simulink model "Hydraulic787"  (R2013a)
settings: Solver=ode23tb  StartTime=0.0  StopTime=1000  RelTol=1e-3
InitFcn:
  | load('SampleOutput.mat')
  | 
  | load('SampleFuelBurn.mat')
undefined symbols (not defined in the file): ailerons, AirProp, B_737, elevator, HydProp, landing_gear, rudder, thrust_rev
libraries: PowerFlowLib x43, simulink x4
(part 1 of 2)
settings Model: Creator=ASELab1  LastModifiedBy=ASELab1
settings SolverCC: SolverJacobianMethodControl=FullAnalytical

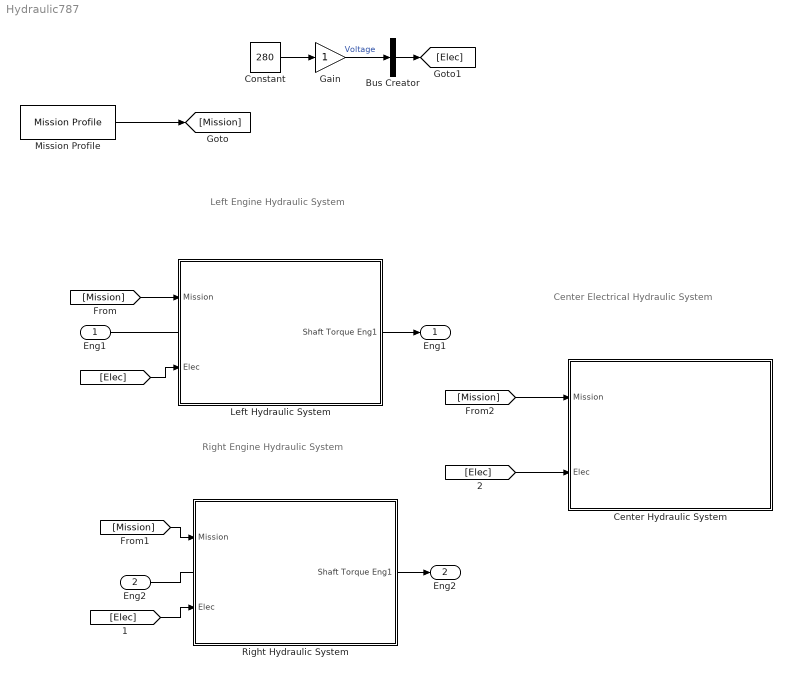
== system Hydraulic787 ==
  note: Left Engine Hydraulic System
  note: Right Engine Hydraulic System
  note: Center Electrical Hydraulic System
  Eng1 : Inport
  Eng2 : Inport  Port=2
  Bus Creator : BusCreator  Inputs=1
  Center Hydraulic System : Subsystem  mask{Hyd_Pump_Pres=34473.79}
      mask prompts: Hyd_Pump_Pres "Hyrdaulic Pump Pressure (kpa)"
  Constant : Constant  Value=280
  Gain : Gain
  Left Hydraulic System : Subsystem  mask{Hyd_Pump_Pres=34473.79}
      mask prompts: Hyd_Pump_Pres "Hyrdaulic Pump Pressure (kpa)"
  Mission Profile : PowerFlowLib/Mission Profile/Mission Profile  mssn_check=off  mssn_prof=MSSN  del_P=0  del_T=0  del_rho=0  pres_msl=101.3  temp_msl=15  dens_msl=1.229
  Right Hydraulic System : Subsystem  mask{Hyd_Pump_Pres=34473.79}
      mask prompts: Hyd_Pump_Pres "Hyrdaulic Pump Pressure (kpa)"
  "Eng1 " : Outport
  "Eng2 " : Outport  Port=2
  wires:
  Mission Profile/1 -> [Mission]
  Eng1/1 -> ?
  [Mission] -> Right Hydraulic System/1(Mission)
  [Mission] -> Center Hydraulic System/1(Mission)
  [Mission] -> Left Hydraulic System/1(Mission)
  Eng2/1 -> ?
  Left Hydraulic System/1(Shaft Torque Eng1) -> "Eng1 "/1
  Right Hydraulic System/1(Shaft Torque Eng1) -> "Eng2 "/1
  [Elec] -> Center Hydraulic System/2(Elec)
  [Elec] -> Left Hydraulic System/2(Elec)
  [Elec] -> Right Hydraulic System/2(Elec)
  Constant/1 -> Gain/1
  Bus Creator/1 -> [Elec]
  Gain/1 -> Bus Creator/1  "Voltage"

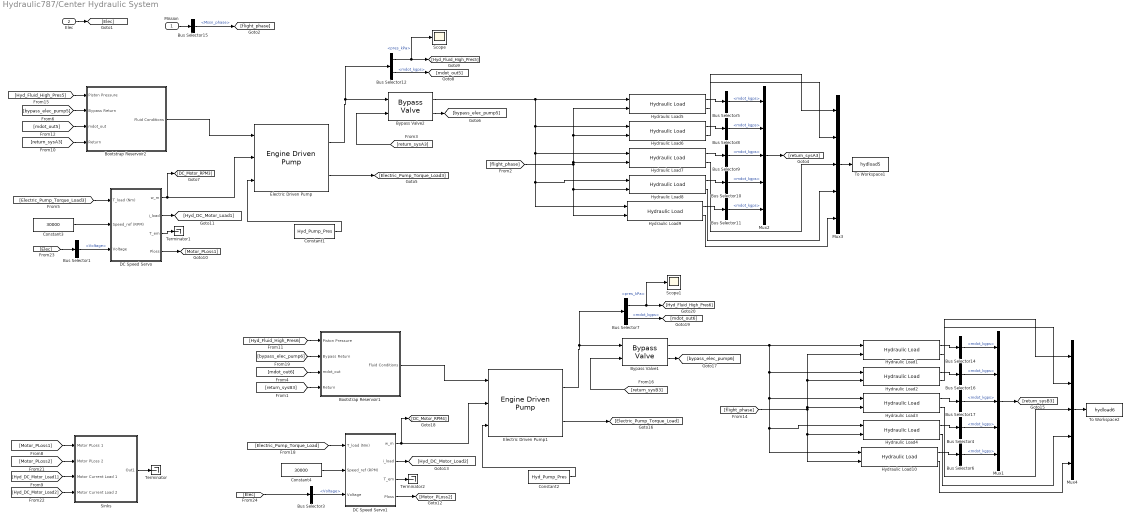
== system Hydraulic787/Center Hydraulic System ==
  Mission : Inport
  Elec : Inport  Port=2
  Bootstrap Reservoir1 : Subsystem  mask(Fluid Reservoir){res_vol=.25, High_Pres_Area=.05, Low_Pres_Area=0, pres_loss=1, T_init=300, P_init=1500, mass_init=30}
      mask prompts: res_vol "Resevoir Volume [m³]"; High_Pres_Area "High Pressure Piston Area"; Low_Pres_Area "Low Pressure Piston Area"; pres_loss "Air Pressure Losses [%]"; T_init "Initial Fluid Temp [K]"; P_init "Initial Air Pressure [kPa]"; mass_init "Initial Fluid Mass [kg]"
      mask help:
      | The fluid reservoir serves as a tank for storing excess hydraulic fluid.
      | The reservoir is fed by returning hydraulic fluid and feeds the engine driven pump.
      | Currently the fluid reservoir tracks the time dependent mass and temperature of the hydraulic fluid in the tank.
      |
      | Block Inputs
      | #1: Bleed air properties (Bus signal)
      | #2: Bypass return from bypass valve
      | #3: Mass flow rate pumped out by hydraulic pump
      | #4: Mass flow rate returned from actuators
      |
      | Block Outputs
      | #1: Bleed air demanded to maintain pressurization
      | #2: Hydraulic fluid properties in the reservoir
      mask init:
      | load AirProp
      | load HydProp
      mask Help: eval('open(''FluidReservoir_help.html'')');
      mask Display:
      | image(imread('hyd_res.png'))
      | 
      | port_label('input',1,'{\bf High Piston Pressure}','TexMode','on')
      | port_label('input',2,'{\bf Bypass Return}','TexMode','on')
      | port_label('input',3,'{\bf m_d_o_t Out}','TexMode','on')
      | port_label('input',4,'{\bf m_d_o_t Return}','TexMode','on')
      | 
      | 
      | port_label('output',1,'{\bf Fluid Out}','TexMode','on')
  Bootstrap Reservoir2 : Subsystem  mask(Fluid Reservoir){res_vol=.25, High_Pres_Area=.05, Low_Pres_Area=0, pres_loss=1, T_init=300, P_init=1500, mass_init=30}
      mask prompts: res_vol "Resevoir Volume [m³]"; High_Pres_Area "High Pressure Piston Area"; Low_Pres_Area "Low Pressure Piston Area"; pres_loss "Air Pressure Losses [%]"; T_init "Initial Fluid Temp [K]"; P_init "Initial Air Pressure [kPa]"; mass_init "Initial Fluid Mass [kg]"
      mask help:
      | The fluid reservoir serves as a tank for storing excess hydraulic fluid.
      | The reservoir is fed by returning hydraulic fluid and feeds the engine driven pump.
      | Currently the fluid reservoir tracks the time dependent mass and temperature of the hydraulic fluid in the tank.
      |
      | Block Inputs
      | #1: Bleed air properties (Bus signal)
      | #2: Bypass return from bypass valve
      | #3: Mass flow rate pumped out by hydraulic pump
      | #4: Mass flow rate returned from actuators
      |
      | Block Outputs
      | #1: Bleed air demanded to maintain pressurization
      | #2: Hydraulic fluid properties in the reservoir
      mask init:
      | load AirProp
      | load HydProp
      mask Help: eval('open(''FluidReservoir_help.html'')');
      mask Display:
      | image(imread('hyd_res.png'))
      | 
      | port_label('input',1,'{\bf High Piston Pressure}','TexMode','on')
      | port_label('input',2,'{\bf Bypass Return}','TexMode','on')
      | port_label('input',3,'{\bf m_d_o_t Out}','TexMode','on')
      | port_label('input',4,'{\bf m_d_o_t Return}','TexMode','on')
      | 
      | 
      | port_label('output',1,'{\bf Fluid Out}','TexMode','on')
  Bus Selector1 : BusSelector  OutputSignals=Voltage
  Bus Selector{4..6,8..11,14,16..17} (10 alike) : BusSelector  OutputSignals=mdot_kgps
  Bus Selector12 : BusSelector  OutputSignals=pres_kPa,mdot_kgps
  Bus Selector15 : BusSelector  OutputSignals=Mssn_phase
  Bus Selector3 : BusSelector  OutputSignals=Voltage
  Bus Selector7 : BusSelector  OutputSignals=pres_kPa,mdot_kgps
  Bypass Valve1 : PowerFlowLib/Energy & Power Systems/Hydraulic/Bypass Valve
  Bypass Valve2 : PowerFlowLib/Energy & Power Systems/Hydraulic/Bypass Valve
  Constant1 : Constant  Value=Hyd_Pump_Pres
  Constant2 : Constant  Value=Hyd_Pump_Pres
  Constant3 : Constant  Value=30000
  Constant4 : Constant  Value=30000
  DC Speed Servo : Subsystem  AncestorBlock=PowerFlowLib/Energy & Power Systems/Electrical/Machines/DC Speed Servo  mask{Vf=390, Ra=0.05, La=0.9e-3, Rfsh=400, Lfsh=320, Lmsh=1.9, J=1.5}
      mask prompts: Vf "Field voltage (V)"; Ra "Armature resistance (Ohms)"; La "Armature inductance (H)"; Rfsh "Shunt field resistance (Ohms)"; Lfsh "Shunt field inductance (H)"; Lmsh "Mutual inductance (H)"; J "Rotor moment of inertia (Kgm^2)"
  DC Speed Servo1 : Subsystem  AncestorBlock=PowerFlowLib/Energy & Power Systems/Electrical/Machines/DC Speed Servo  mask{Vf=390, Ra=0.05, La=0.9e-3, Rfsh=400, Lfsh=320, Lmsh=1.9, J=1.5}
      mask prompts: Vf "Field voltage (V)"; Ra "Armature resistance (Ohms)"; La "Armature inductance (H)"; Rfsh "Shunt field resistance (Ohms)"; Lfsh "Shunt field inductance (H)"; Lmsh "Mutual inductance (H)"; J "Rotor moment of inertia (Kgm^2)"
  Electric Driven Pump : PowerFlowLib/Energy & Power Systems/Hydraulic/Engine Driven Pump  RPM=3750  disp=39  eta_mech=95  eta_v=85  nom_T=40  nom_w=393  nom_delP=20684
  Electric Driven Pump1 : PowerFlowLib/Energy & Power Systems/Hydraulic/Engine Driven Pump  RPM=3750  disp=39  eta_mech=95  eta_v=85  nom_T=40  nom_w=393  nom_delP=20684
  Hydraulic Load1 : PowerFlowLib/Energy & Power Systems/Hydraulic/Hydraulic Load  fileslct=off  filename=HydraulicLoad.mat  filedir=C:\Users\mwillms4\Dropbox\School\Graduate\Research\PowerFlow Development\PowerFlow Summer 2013\PropertyTables\HydraulicLoad.mat  var_struct=HydraulicLoad  h_load=B_737 - rudder
  Hydraulic Load10 : PowerFlowLib/Energy & Power Systems/Hydraulic/Hydraulic Load  fileslct=off  filename=HydraulicLoad.mat  filedir=C:\Users\mwillms4\Dropbox\School\Graduate\Research\PowerFlow Development\PowerFlow Summer 2013\PropertyTables\HydraulicLoad.mat  var_struct=HydraulicLoad  h_load=B_737 - thrust_rev
  Hydraulic Load2 : PowerFlowLib/Energy & Power Systems/Hydraulic/Hydraulic Load  fileslct=off  filename=HydraulicLoad.mat  filedir=C:\Users\mwillms4\Dropbox\School\Graduate\Research\PowerFlow Development\PowerFlow Summer 2013\PropertyTables\HydraulicLoad.mat  var_struct=HydraulicLoad  h_load=B_737 - ailerons
  Hydraulic Load3 : PowerFlowLib/Energy & Power Systems/Hydraulic/Hydraulic Load  fileslct=off  filename=HydraulicLoad.mat  filedir=C:\Users\mwillms4\Dropbox\School\Graduate\Research\PowerFlow Development\PowerFlow Summer 2013\PropertyTables\HydraulicLoad.mat  var_struct=HydraulicLoad  h_load=B_737 - elevator
  Hydraulic Load4 : PowerFlowLib/Energy & Power Systems/Hydraulic/Hydraulic Load  fileslct=off  filename=HydraulicLoad.mat  filedir=C:\Users\mwillms4\Dropbox\School\Graduate\Research\PowerFlow Development\PowerFlow Summer 2013\PropertyTables\HydraulicLoad.mat  var_struct=HydraulicLoad  h_load=B_737 - landing_gear
  Hydraulic Load5 : PowerFlowLib/Energy & Power Systems/Hydraulic/Hydraulic Load  fileslct=off  filename=HydraulicLoad.mat  filedir=C:\Users\mwillms4\Dropbox\School\Graduate\Research\PowerFlow Development\PowerFlow Summer 2013\PropertyTables\HydraulicLoad.mat  var_struct=HydraulicLoad  h_load=B_737 - rudder
  Hydraulic Load6 : PowerFlowLib/Energy & Power Systems/Hydraulic/Hydraulic Load  fileslct=off  filename=HydraulicLoad.mat  filedir=C:\Users\mwillms4\Dropbox\School\Graduate\Research\PowerFlow Development\PowerFlow Summer 2013\PropertyTables\HydraulicLoad.mat  var_struct=HydraulicLoad  h_load=B_737 - ailerons
  Hydraulic Load7 : PowerFlowLib/Energy & Power Systems/Hydraulic/Hydraulic Load  fileslct=off  filename=HydraulicLoad.mat  filedir=C:\Users\mwillms4\Dropbox\School\Graduate\Research\PowerFlow Development\PowerFlow Summer 2013\PropertyTables\HydraulicLoad.mat  var_struct=HydraulicLoad  h_load=B_737 - elevator
  Hydraulic Load8 : PowerFlowLib/Energy & Power Systems/Hydraulic/Hydraulic Load  fileslct=off  filename=HydraulicLoad.mat  filedir=C:\Users\mwillms4\Dropbox\School\Graduate\Research\PowerFlow Development\PowerFlow Summer 2013\PropertyTables\HydraulicLoad.mat  var_struct=HydraulicLoad  h_load=B_737 - landing_gear
  Hydraulic Load9 : PowerFlowLib/Energy & Power Systems/Hydraulic/Hydraulic Load  fileslct=off  filename=HydraulicLoad.mat  filedir=C:\Users\mwillms4\Dropbox\School\Graduate\Research\PowerFlow Development\PowerFlow Summer 2013\PropertyTables\HydraulicLoad.mat  var_struct=HydraulicLoad  h_load=B_737 - thrust_rev
  Mux{1..4} (4 alike) : Mux  Inputs=5
  Scope : Scope
  Scope1 : Scope
      settings: SaveName=ScopeData2
  Sinks : Subsystem
  Terminator : Terminator
  Terminator1 : Terminator
  Terminator2 : Terminator
  To Workspace1 : ToWorkspace  VariableName=hydload5  SampleTime=10  SaveFormat=Structure With Time
  To Workspace2 : ToWorkspace  VariableName=hydload6  SampleTime=10  SaveFormat=Structure With Time
  wires:
  Bus Selector15/1 -> [flight_phase]  "<Mssn_phase>"
  Mission/1 -> Bus Selector15/1
  DC Speed Servo/1(w_m) -> Electric Driven Pump/2, [DC_Motor_RPM3]
  Bus Selector1/1 -> DC Speed Servo/3(Voltage)  "<Voltage>"
  Hydraulic Load5/1 -> Bus Selector5/1
  Bypass Valve2/1 -> Hydraulic Load9/1, Hydraulic Load8/1, Hydraulic Load7/1, Hydraulic Load6/1, Hydraulic Load5/1
  Hydraulic Load6/2 -> Mux3/2
  Hydraulic Load7/2 -> Mux3/3
  Hydraulic Load6/1 -> Bus Selector8/1
  Hydraulic Load7/1 -> Bus Selector9/1
  Bus Selector8/1 -> Mux2/2  "<mdot_kgps>"
  Bus Selector5/1 -> Mux2/1  "<mdot_kgps>"
  Bus Selector9/1 -> Mux2/3  "<mdot_kgps>"
  Mux2/1 -> [return_sysA3]
  [flight_phase] -> Hydraulic Load9/2, Hydraulic Load8/2, Hydraulic Load5/2, Hydraulic Load6/2, Hydraulic Load7/2
  Hydraulic Load8/1 -> Bus Selector10/1
  Hydraulic Load9/1 -> Bus Selector11/1
  Hydraulic Load9/2 -> Mux3/5
  Hydraulic Load8/2 -> Mux3/4
  Bus Selector10/1 -> Mux2/4  "<mdot_kgps>"
  Bus Selector11/1 -> Mux2/5  "<mdot_kgps>"
  Hydraulic Load5/2 -> Mux3/1
  Mux3/1 -> To Workspace1/1
  Electric Driven Pump/1 -> Bus Selector12/1, Bypass Valve2/1
  [return_sysA3] -> Bypass Valve2/2
  Constant1/1 -> Electric Driven Pump/3
  Electric Driven Pump/2 -> [Electric_Pump_Torque_Load3]
  [Electric_Pump_Torque_Load3] -> DC Speed Servo/1(T_load (Nm))
  Bypass Valve2/2 -> [bypass_elec_pump5]
  [bypass_elec_pump5] -> Bootstrap Reservoir2/2(Bypass Return)
  Bootstrap Reservoir2/1(Fluid Conditions) -> Electric Driven Pump/1
  Constant3/1 -> DC Speed Servo/2(Speed_ref (RPM))
  Bus Selector12/1 -> Scope/1, [Hyd_Fluid_High_Pres5]  "<pres_kPa>"
  Bus Selector12/2 -> [mdot_out5]  "<mdot_kgps>"
  DC Speed Servo/4(Ploss) -> [Motor_PLoss1]
  [Motor_PLoss1] -> Sinks/1("Motor PLoss 1 ")
  DC Speed Servo/2(i_load) -> [Hyd_DC_Motor_Load1]
  [Hyd_DC_Motor_Load1] -> Sinks/3(Motor Current Load 1)
  [return_sysA3] -> Bootstrap Reservoir2/4(Return)
  [mdot_out5] -> Bootstrap Reservoir2/3(mdot_out)
  [Hyd_Fluid_High_Pres5] -> Bootstrap Reservoir2/1(Piston Pressure)
  DC Speed Servo1/1(w_m) -> Electric Driven Pump1/2, [DC_Motor_RPM4]
  [Elec] -> Bus Selector3/1
  Bus Selector3/1 -> DC Speed Servo1/3(Voltage)  "<Voltage>"
  Hydraulic Load1/1 -> Bus Selector14/1
  Bypass Valve1/1 -> Hydraulic Load10/1, Hydraulic Load4/1, Hydraulic Load3/1, Hydraulic Load2/1, Hydraulic Load1/1
  Hydraulic Load2/2 -> Mux4/2
  Hydraulic Load3/2 -> Mux4/3
  Hydraulic Load2/1 -> Bus Selector16/1
  Hydraulic Load3/1 -> Bus Selector17/1
  Bus Selector16/1 -> Mux1/2  "<mdot_kgps>"
  Bus Selector14/1 -> Mux1/1  "<mdot_kgps>"
  Bus Selector17/1 -> Mux1/3  "<mdot_kgps>"
  Mux1/1 -> [return_sysB3]
  [flight_phase] -> Hydraulic Load10/2, Hydraulic Load4/2, Hydraulic Load1/2, Hydraulic Load2/2, Hydraulic Load3/2
  Hydraulic Load4/1 -> Bus Selector4/1
  Hydraulic Load10/1 -> Bus Selector6/1
  Hydraulic Load10/2 -> Mux4/5
  Hydraulic Load4/2 -> Mux4/4
  Bus Selector4/1 -> Mux1/4  "<mdot_kgps>"
  Bus Selector6/1 -> Mux1/5  "<mdot_kgps>"
  Hydraulic Load1/2 -> Mux4/1
  Mux4/1 -> To Workspace2/1
  Electric Driven Pump1/1 -> Bus Selector7/1, Bypass Valve1/1
  [return_sysB3] -> Bypass Valve1/2
  Constant2/1 -> Electric Driven Pump1/3
  Electric Driven Pump1/2 -> [Electric_Pump_Torque_Load]
  [Electric_Pump_Torque_Load] -> DC Speed Servo1/1(T_load (Nm))
  Bypass Valve1/2 -> [bypass_elec_pump6]
  [bypass_elec_pump6] -> Bootstrap Reservoir1/2(Bypass Return)
  Bootstrap Reservoir1/1(Fluid Conditions) -> Electric Driven Pump1/1
  Constant4/1 -> DC Speed Servo1/2(Speed_ref (RPM))
  Bus Selector7/1 -> Scope1/1, [Hyd_Fluid_High_Pres6]  "<pres_kPa>"
  Bus Selector7/2 -> [mdot_out6]  "<mdot_kgps>"
  DC Speed Servo1/4(Ploss) -> [Motor_PLoss2]
  DC Speed Servo1/2(i_load) -> [Hyd_DC_Motor_Load2]
  [return_sysB3] -> Bootstrap Reservoir1/4(Return)
  [mdot_out6] -> Bootstrap Reservoir1/3(mdot_out)
  [Hyd_Fluid_High_Pres6] -> Bootstrap Reservoir1/1(Piston Pressure)
  [Motor_PLoss2] -> Sinks/2(Motor PLoss 2)
  [Hyd_DC_Motor_Load2] -> Sinks/4(Motor Current Load 2)
  [Elec] -> Bus Selector1/1
  Elec/1 -> [Elec]
  Sinks/1(Out1) -> Terminator/1
  DC Speed Servo1/3(T_em) -> Terminator2/1
  DC Speed Servo/3(T_em) -> Terminator1/1

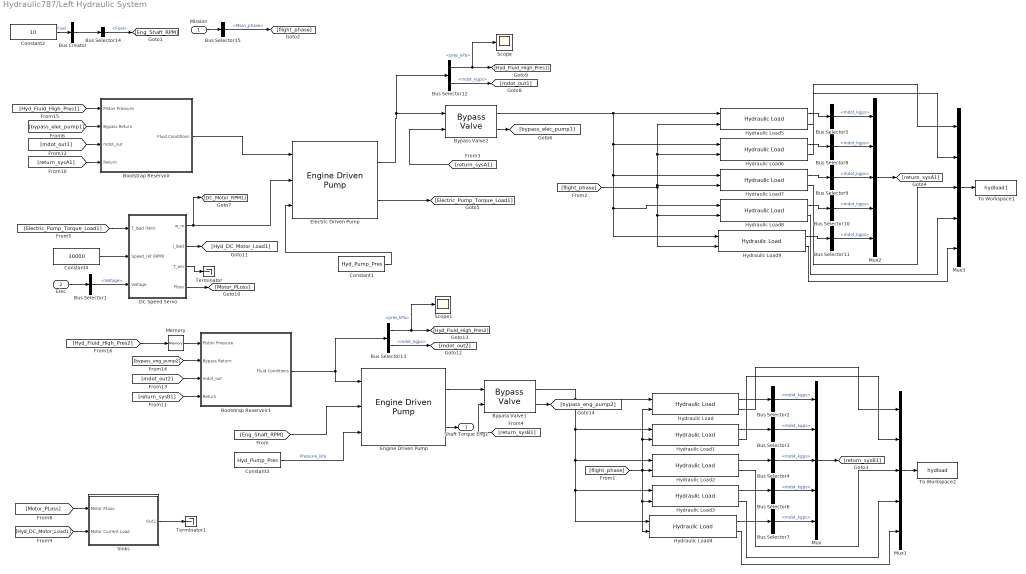
== system Hydraulic787/Left Hydraulic System ==
  Mission : Inport
  Elec : Inport  Port=2
  Bootstrap Reservoir : Subsystem  mask(Fluid Reservoir){res_vol=.25, High_Pres_Area=.05, Low_Pres_Area=0, pres_loss=1, T_init=300, P_init=1500, mass_init=30}
      mask prompts: res_vol "Resevoir Volume [m³]"; High_Pres_Area "High Pressure Piston Area"; Low_Pres_Area "Low Pressure Piston Area"; pres_loss "Air Pressure Losses [%]"; T_init "Initial Fluid Temp [K]"; P_init "Initial Air Pressure [kPa]"; mass_init "Initial Fluid Mass [kg]"
      mask help:
      | The fluid reservoir serves as a tank for storing excess hydraulic fluid.
      | The reservoir is fed by returning hydraulic fluid and feeds the engine driven pump.
      | Currently the fluid reservoir tracks the time dependent mass and temperature of the hydraulic fluid in the tank.
      |
      | Block Inputs
      | #1: Bleed air properties (Bus signal)
      | #2: Bypass return from bypass valve
      | #3: Mass flow rate pumped out by hydraulic pump
      | #4: Mass flow rate returned from actuators
      |
      | Block Outputs
      | #1: Bleed air demanded to maintain pressurization
      | #2: Hydraulic fluid properties in the reservoir
      mask init:
      | load AirProp
      | load HydProp
      mask Help: eval('open(''FluidReservoir_help.html'')');
      mask Display:
      | image(imread('hyd_res.png'))
      | 
      | port_label('input',1,'{\bf High Piston Pressure}','TexMode','on')
      | port_label('input',2,'{\bf Bypass Return}','TexMode','on')
      | port_label('input',3,'{\bf m_d_o_t Out}','TexMode','on')
      | port_label('input',4,'{\bf m_d_o_t Return}','TexMode','on')
      | 
      | 
      | port_label('output',1,'{\bf Fluid Out}','TexMode','on')
  Bootstrap Reservoir1 : Subsystem  mask(Fluid Reservoir){res_vol=.25, High_Pres_Area=.05, Low_Pres_Area=0, pres_loss=1, T_init=300, P_init=1500, mass_init=30}
      mask prompts: res_vol "Resevoir Volume [m³]"; High_Pres_Area "High Pressure Piston Area"; Low_Pres_Area "Low Pressure Piston Area"; pres_loss "Air Pressure Losses [%]"; T_init "Initial Fluid Temp [K]"; P_init "Initial Air Pressure [kPa]"; mass_init "Initial Fluid Mass [kg]"
      mask help:
      | The fluid reservoir serves as a tank for storing excess hydraulic fluid.
      | The reservoir is fed by returning hydraulic fluid and feeds the engine driven pump.
      | Currently the fluid reservoir tracks the time dependent mass and temperature of the hydraulic fluid in the tank.
      |
      | Block Inputs
      | #1: Bleed air properties (Bus signal)
      | #2: Bypass return from bypass valve
      | #3: Mass flow rate pumped out by hydraulic pump
      | #4: Mass flow rate returned from actuators
      |
      | Block Outputs
      | #1: Bleed air demanded to maintain pressurization
      | #2: Hydraulic fluid properties in the reservoir
      mask init:
      | load AirProp
      | load HydProp
      mask Help: eval('open(''FluidReservoir_help.html'')');
      mask Display:
      | image(imread('hyd_res.png'))
      | 
      | port_label('input',1,'{\bf High Piston Pressure}','TexMode','on')
      | port_label('input',2,'{\bf Bypass Return}','TexMode','on')
      | port_label('input',3,'{\bf m_d_o_t Out}','TexMode','on')
      | port_label('input',4,'{\bf m_d_o_t Return}','TexMode','on')
      | 
      | 
      | port_label('output',1,'{\bf Fluid Out}','TexMode','on')
  Bus Creator : BusCreator  Inputs=1
  Bus Selector1 : BusSelector  OutputSignals=Voltage
  Bus Selector{2..11} (10 alike) : BusSelector  OutputSignals=mdot_kgps
  Bus Selector12 : BusSelector  OutputSignals=pres_kPa,mdot_kgps
  Bus Selector13 : BusSelector  OutputSignals=pres_kPa,mdot_kgps
  Bus Selector14 : BusSelector  OutputSignals=Fuel
  Bus Selector15 : BusSelector  OutputSignals=Mssn_phase
  Bypass Valve1 : PowerFlowLib/Energy & Power Systems/Hydraulic/Bypass Valve
  Bypass Valve2 : PowerFlowLib/Energy & Power Systems/Hydraulic/Bypass Valve
  Constant1 : Constant  Value=Hyd_Pump_Pres
  Constant2 : Constant  Value=10
  Constant3 : Constant  Value=Hyd_Pump_Pres
  Constant4 : Constant  Value=30000
  DC Speed Servo : Subsystem  AncestorBlock=PowerFlowLib/Energy & Power Systems/Electrical/Machines/DC Speed Servo  mask{Vf=280, Ra=0.05, La=0.9e-3, Rfsh=400, Lfsh=320, Lmsh=1.9, J=1.5}
      mask prompts: Vf "Field voltage (V)"; Ra "Armature resistance (Ohms)"; La "Armature inductance (H)"; Rfsh "Shunt field resistance (Ohms)"; Lfsh "Shunt field inductance (H)"; Lmsh "Mutual inductance (H)"; J "Rotor moment of inertia (Kgm^2)"
  Electric Driven Pump : PowerFlowLib/Energy & Power Systems/Hydraulic/Engine Driven Pump  RPM=3750  disp=39  eta_mech=95  eta_v=85  nom_T=40  nom_w=393  nom_delP=20684
  Engine Driven Pump : PowerFlowLib/Energy & Power Systems/Hydraulic/Engine Driven Pump  RPM=3750  disp=39  eta_mech=95  eta_v=85  nom_T=40  nom_w=393  nom_delP=20684
  Hydraulic Load : PowerFlowLib/Energy & Power Systems/Hydraulic/Hydraulic Load  fileslct=off  filename=HydraulicLoad.mat  filedir=C:\Users\mwillms4\Dropbox\School\Graduate\Research\PowerFlow Development\PowerFlow Summer 2013\PropertyTables\HydraulicLoad.mat  var_struct=HydraulicLoad  h_load=B_737 - rudder
  Hydraulic Load1 : PowerFlowLib/Energy & Power Systems/Hydraulic/Hydraulic Load  fileslct=off  filename=HydraulicLoad.mat  filedir=C:\Users\mwillms4\Dropbox\School\Graduate\Research\PowerFlow Development\PowerFlow Summer 2013\PropertyTables\HydraulicLoad.mat  var_struct=HydraulicLoad  h_load=B_737 - ailerons
  Hydraulic Load2 : PowerFlowLib/Energy & Power Systems/Hydraulic/Hydraulic Load  fileslct=off  filename=HydraulicLoad.mat  filedir=C:\Users\mwillms4\Dropbox\School\Graduate\Research\PowerFlow Development\PowerFlow Summer 2013\PropertyTables\HydraulicLoad.mat  var_struct=HydraulicLoad  h_load=B_737 - elevator
  Hydraulic Load3 : PowerFlowLib/Energy & Power Systems/Hydraulic/Hydraulic Load  fileslct=off  filename=HydraulicLoad.mat  filedir=C:\Users\mwillms4\Dropbox\School\Graduate\Research\PowerFlow Development\PowerFlow Summer 2013\PropertyTables\HydraulicLoad.mat  var_struct=HydraulicLoad  h_load=B_737 - landing_gear
  Hydraulic Load4 : PowerFlowLib/Energy & Power Systems/Hydraulic/Hydraulic Load  fileslct=off  filename=HydraulicLoad.mat  filedir=C:\Users\mwillms4\Dropbox\School\Graduate\Research\PowerFlow Development\PowerFlow Summer 2013\PropertyTables\HydraulicLoad.mat  var_struct=HydraulicLoad  h_load=B_737 - thrust_rev
  Hydraulic Load5 : PowerFlowLib/Energy & Power Systems/Hydraulic/Hydraulic Load  fileslct=off  filename=HydraulicLoad.mat  filedir=C:\Users\mwillms4\Dropbox\School\Graduate\Research\PowerFlow Development\PowerFlow Summer 2013\PropertyTables\HydraulicLoad.mat  var_struct=HydraulicLoad  h_load=B_737 - rudder
  Hydraulic Load6 : PowerFlowLib/Energy & Power Systems/Hydraulic/Hydraulic Load  fileslct=off  filename=HydraulicLoad.mat  filedir=C:\Users\mwillms4\Dropbox\School\Graduate\Research\PowerFlow Development\PowerFlow Summer 2013\PropertyTables\HydraulicLoad.mat  var_struct=HydraulicLoad  h_load=B_737 - ailerons
  Hydraulic Load7 : PowerFlowLib/Energy & Power Systems/Hydraulic/Hydraulic Load  fileslct=off  filename=HydraulicLoad.mat  filedir=C:\Users\mwillms4\Dropbox\School\Graduate\Research\PowerFlow Development\PowerFlow Summer 2013\PropertyTables\HydraulicLoad.mat  var_struct=HydraulicLoad  h_load=B_737 - elevator
  Hydraulic Load8 : PowerFlowLib/Energy & Power Systems/Hydraulic/Hydraulic Load  fileslct=off  filename=HydraulicLoad.mat  filedir=C:\Users\mwillms4\Dropbox\School\Graduate\Research\PowerFlow Development\PowerFlow Summer 2013\PropertyTables\HydraulicLoad.mat  var_struct=HydraulicLoad  h_load=B_737 - landing_gear
  Hydraulic Load9 : PowerFlowLib/Energy & Power Systems/Hydraulic/Hydraulic Load  fileslct=off  filename=HydraulicLoad.mat  filedir=C:\Users\mwillms4\Dropbox\School\Graduate\Research\PowerFlow Development\PowerFlow Summer 2013\PropertyTables\HydraulicLoad.mat  var_struct=HydraulicLoad  h_load=B_737 - thrust_rev
  Memory : Memory
  Mux{,1..3} (4 alike) : Mux  Inputs=5
  Scope : Scope
  Scope1 : Scope
  Sinks : Subsystem
  Terminator : Terminator
  Terminator1 : Terminator
  To Workspace1 : ToWorkspace  VariableName=hydload1  SampleTime=10  SaveFormat=Structure With Time
  To Workspace2 : ToWorkspace  VariableName=hydload  SampleTime=10  SaveFormat=Structure With Time
  Shaft Torque Eng1 : Outport
  wires:
  Bus Selector15/1 -> [flight_phase]  "<Mssn_phase>"
  Mission/1 -> Bus Selector15/1
  DC Speed Servo/1(w_m) -> Electric Driven Pump/2, [DC_Motor_RPM1]
  Constant3/1 -> Engine Driven Pump/3  "Pressure_kPa"
  Constant2/1 -> Bus Creator/1  "Fuel"
  [Eng_Shaft_RPM] -> Engine Driven Pump/2
  Elec/1 -> Bus Selector1/1
  Bus Selector1/1 -> DC Speed Servo/3(Voltage)  "<Voltage>"
  Engine Driven Pump/2 -> Shaft Torque Eng1/1
  Hydraulic Load/1 -> Bus Selector2/1
  Bypass Valve1/1 -> Hydraulic Load3/1, Hydraulic Load4/1, Hydraulic Load2/1, Hydraulic Load1/1, Hydraulic Load/1
  Hydraulic Load1/2 -> Mux1/2
  Hydraulic Load2/2 -> Mux1/3
  Hydraulic Load1/1 -> Bus Selector3/1
  Hydraulic Load2/1 -> Bus Selector4/1
  Bus Selector3/1 -> Mux/2  "<mdot_kgps>"
  Bus Selector2/1 -> Mux/1  "<mdot_kgps>"
  Bus Selector4/1 -> Mux/3  "<mdot_kgps>"
  Mux/1 -> [return_sysB1]
  [flight_phase] -> Hydraulic Load/2, Hydraulic Load1/2, Hydraulic Load3/2, Hydraulic Load4/2, Hydraulic Load2/2
  Hydraulic Load3/1 -> Bus Selector6/1
  Hydraulic Load4/1 -> Bus Selector7/1
  Hydraulic Load4/2 -> Mux1/5
  Hydraulic Load3/2 -> Mux1/4
  Bus Selector6/1 -> Mux/4  "<mdot_kgps>"
  Bus Selector7/1 -> Mux/5  "<mdot_kgps>"
  Hydraulic Load/2 -> Mux1/1
  Mux1/1 -> To Workspace2/1
  Hydraulic Load5/1 -> Bus Selector5/1
  Bypass Valve2/1 -> Hydraulic Load9/1, Hydraulic Load8/1, Hydraulic Load7/1, Hydraulic Load6/1, Hydraulic Load5/1
  Hydraulic Load6/2 -> Mux3/2
  Hydraulic Load7/2 -> Mux3/3
  Hydraulic Load6/1 -> Bus Selector8/1
  Hydraulic Load7/1 -> Bus Selector9/1
  Bus Selector8/1 -> Mux2/2  "<mdot_kgps>"
  Bus Selector5/1 -> Mux2/1  "<mdot_kgps>"
  Bus Selector9/1 -> Mux2/3  "<mdot_kgps>"
  Mux2/1 -> [return_sysA1]
  [flight_phase] -> Hydraulic Load9/2, Hydraulic Load8/2, Hydraulic Load5/2, Hydraulic Load6/2, Hydraulic Load7/2
  Hydraulic Load8/1 -> Bus Selector10/1
  Hydraulic Load9/1 -> Bus Selector11/1
  Hydraulic Load9/2 -> Mux3/5
  Hydraulic Load8/2 -> Mux3/4
  Bus Selector10/1 -> Mux2/4  "<mdot_kgps>"
  Bus Selector11/1 -> Mux2/5  "<mdot_kgps>"
  Hydraulic Load5/2 -> Mux3/1
  Mux3/1 -> To Workspace1/1
  Engine Driven Pump/1 -> Bypass Valve1/1
  Electric Driven Pump/1 -> Bus Selector12/1, Bypass Valve2/1
  [return_sysA1] -> Bypass Valve2/2
  [return_sysB1] -> Bypass Valve1/2
  Constant1/1 -> Electric Driven Pump/3
  Electric Driven Pump/2 -> [Electric_Pump_Torque_Load1]
  [Electric_Pump_Torque_Load1] -> DC Speed Servo/1(T_load (Nm))
  Bypass Valve2/2 -> [bypass_elec_pump1]
  [bypass_elec_pump1] -> Bootstrap Reservoir/2(Bypass Return)
  Bootstrap Reservoir/1(Fluid Conditions) -> Electric Driven Pump/1
  Constant4/1 -> DC Speed Servo/2(Speed_ref (RPM))
  Bus Selector12/1 -> Scope/1, [Hyd_Fluid_High_Pres1]  "<pres_kPa>"
  Bus Selector12/2 -> [mdot_out1]  "<mdot_kgps>"
  DC Speed Servo/4(Ploss) -> [Motor_PLoss]
  [Motor_PLoss] -> Sinks/1("Motor PLoss ")
  DC Speed Servo/2(i_load) -> [Hyd_DC_Motor_Load1]
  [Hyd_DC_Motor_Load1] -> Sinks/2(Motor Current Load)
  Bootstrap Reservoir1/1(Fluid Conditions) -> Engine Driven Pump/1, Bus Selector13/1
  Bus Selector13/1 -> Scope1/1, [Hyd_Fluid_High_Pres2]  "<pres_kPa>"
  Bus Selector13/2 -> [mdot_out2]  "<mdot_kgps>"
  [return_sysA1] -> Bootstrap Reservoir/4(Return)
  [return_sysB1] -> Bootstrap Reservoir1/4(Return)
  [mdot_out1] -> Bootstrap Reservoir/3(mdot_out)
  Bypass Valve1/2 -> [bypass_eng_pump2]
  [bypass_eng_pump2] -> Bootstrap Reservoir1/2(Bypass Return)
  [mdot_out2] -> Bootstrap Reservoir1/3(mdot_out)
  [Hyd_Fluid_High_Pres1] -> Bootstrap Reservoir/1(Piston Pressure)
  [Hyd_Fluid_High_Pres2] -> Memory/1
  Bus Selector14/1 -> [Eng_Shaft_RPM]  "<Fuel>"
  Bus Creator/1 -> Bus Selector14/1
  DC Speed Servo/3(T_em) -> Terminator/1
  Sinks/1(Out1) -> Terminator1/1
  Memory/1 -> Bootstrap Reservoir1/1(Piston Pressure)

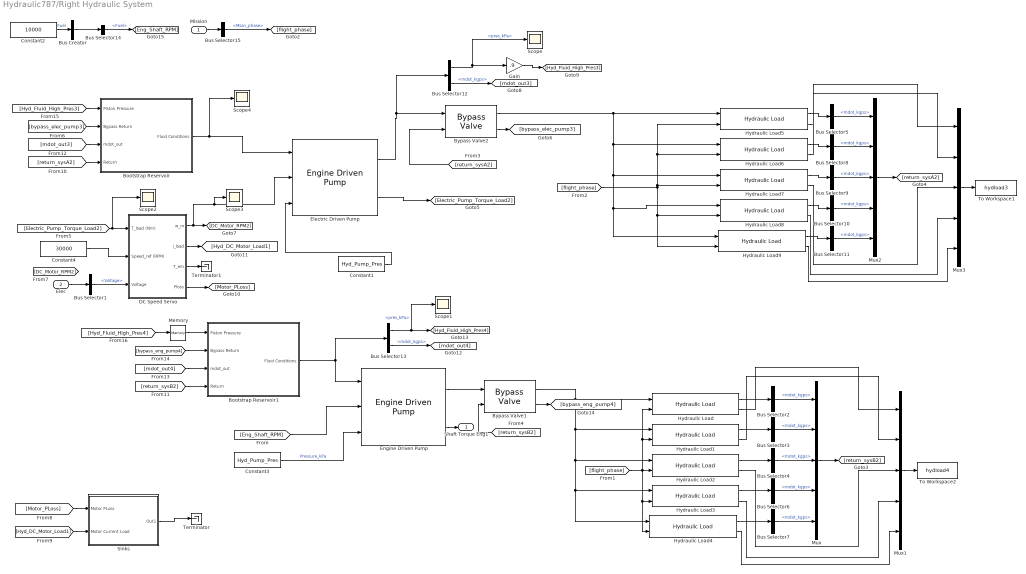
== system Hydraulic787/Right Hydraulic System ==
  Mission : Inport
  Elec : Inport  Port=2
  Bootstrap Reservoir : Subsystem  mask(Fluid Reservoir){res_vol=.25, High_Pres_Area=.05, Low_Pres_Area=0, pres_loss=1, T_init=300, P_init=1500, mass_init=30}
      mask prompts: res_vol "Resevoir Volume [m³]"; High_Pres_Area "High Pressure Piston Area"; Low_Pres_Area "Low Pressure Piston Area"; pres_loss "Air Pressure Losses [%]"; T_init "Initial Fluid Temp [K]"; P_init "Initial Air Pressure [kPa]"; mass_init "Initial Fluid Mass [kg]"
      mask help:
      | The fluid reservoir serves as a tank for storing excess hydraulic fluid.
      | The reservoir is fed by returning hydraulic fluid and feeds the engine driven pump.
      | Currently the fluid reservoir tracks the time dependent mass and temperature of the hydraulic fluid in the tank.
      |
      | Block Inputs
      | #1: Bleed air properties (Bus signal)
      | #2: Bypass return from bypass valve
      | #3: Mass flow rate pumped out by hydraulic pump
      | #4: Mass flow rate returned from actuators
      |
      | Block Outputs
      | #1: Bleed air demanded to maintain pressurization
      | #2: Hydraulic fluid properties in the reservoir
      mask init:
      | load AirProp
      | load HydProp
      mask Help: eval('open(''FluidReservoir_help.html'')');
      mask Display:
      | image(imread('hyd_res.png'))
      | 
      | port_label('input',1,'{\bf High Piston Pressure}','TexMode','on')
      | port_label('input',2,'{\bf Bypass Return}','TexMode','on')
      | port_label('input',3,'{\bf m_d_o_t Out}','TexMode','on')
      | port_label('input',4,'{\bf m_d_o_t Return}','TexMode','on')
      | 
      | 
      | port_label('output',1,'{\bf Fluid Out}','TexMode','on')
  Bootstrap Reservoir1 : Subsystem  mask(Fluid Reservoir){res_vol=.25, High_Pres_Area=.05, Low_Pres_Area=0, pres_loss=1, T_init=300, P_init=1500, mass_init=30}
      mask prompts: res_vol "Resevoir Volume [m³]"; High_Pres_Area "High Pressure Piston Area"; Low_Pres_Area "Low Pressure Piston Area"; pres_loss "Air Pressure Losses [%]"; T_init "Initial Fluid Temp [K]"; P_init "Initial Air Pressure [kPa]"; mass_init "Initial Fluid Mass [kg]"
      mask help:
      | The fluid reservoir serves as a tank for storing excess hydraulic fluid.
      | The reservoir is fed by returning hydraulic fluid and feeds the engine driven pump.
      | Currently the fluid reservoir tracks the time dependent mass and temperature of the hydraulic fluid in the tank.
      |
      | Block Inputs
      | #1: Bleed air properties (Bus signal)
      | #2: Bypass return from bypass valve
      | #3: Mass flow rate pumped out by hydraulic pump
      | #4: Mass flow rate returned from actuators
      |
      | Block Outputs
      | #1: Bleed air demanded to maintain pressurization
      | #2: Hydraulic fluid properties in the reservoir
      mask init:
      | load AirProp
      | load HydProp
      mask Help: eval('open(''FluidReservoir_help.html'')');
      mask Display:
      | image(imread('hyd_res.png'))
      | 
      | port_label('input',1,'{\bf High Piston Pressure}','TexMode','on')
      | port_label('input',2,'{\bf Bypass Return}','TexMode','on')
      | port_label('input',3,'{\bf m_d_o_t Out}','TexMode','on')
      | port_label('input',4,'{\bf m_d_o_t Return}','TexMode','on')
      | 
      | 
      | port_label('output',1,'{\bf Fluid Out}','TexMode','on')
  Bus Creator : BusCreator  Inputs=1
  Bus Selector1 : BusSelector  OutputSignals=Voltage
  Bus Selector{2..11} (10 alike) : BusSelector  OutputSignals=mdot_kgps
  Bus Selector12 : BusSelector  OutputSignals=pres_kPa,mdot_kgps
  Bus Selector13 : BusSelector  OutputSignals=pres_kPa,mdot_kgps
  Bus Selector14 : BusSelector  OutputSignals=Fuel
  Bus Selector15 : BusSelector  OutputSignals=Mssn_phase
  Bypass Valve1 : PowerFlowLib/Energy & Power Systems/Hydraulic/Bypass Valve
  Bypass Valve2 : PowerFlowLib/Energy & Power Systems/Hydraulic/Bypass Valve
  Constant1 : Constant  Value=Hyd_Pump_Pres
  Constant2 : Constant  Value=10000
  Constant3 : Constant  Value=Hyd_Pump_Pres
  Constant4 : Constant  Value=30000
  DC Speed Servo : Subsystem  AncestorBlock=PowerFlowLib/Energy & Power Systems/Electrical/Machines/DC Speed Servo  mask{Vf=390, Ra=0.05, La=0.9e-3, Rfsh=400, Lfsh=320, Lmsh=1.9, J=1.5}
      mask prompts: Vf "Field voltage (V)"; Ra "Armature resistance (Ohms)"; La "Armature inductance (H)"; Rfsh "Shunt field resistance (Ohms)"; Lfsh "Shunt field inductance (H)"; Lmsh "Mutual inductance (H)"; J "Rotor moment of inertia (Kgm^2)"
  Electric Driven Pump : PowerFlowLib/Energy & Power Systems/Hydraulic/Engine Driven Pump  RPM=3750  disp=39  eta_mech=95  eta_v=85  nom_T=40  nom_w=393  nom_delP=20684
  Engine Driven Pump : PowerFlowLib/Energy & Power Systems/Hydraulic/Engine Driven Pump  RPM=3750  disp=39  eta_mech=95  eta_v=85  nom_T=40  nom_w=393  nom_delP=20684
  Gain : Gain  Gain=.9
  Hydraulic Load : PowerFlowLib/Energy & Power Systems/Hydraulic/Hydraulic Load  fileslct=off  filename=HydraulicLoad.mat  filedir=C:\Users\mwillms4\Dropbox\School\Graduate\Research\PowerFlow Development\PowerFlow Summer 2013\PropertyTables\HydraulicLoad.mat  var_struct=HydraulicLoad  h_load=B_737 - rudder
  Hydraulic Load1 : PowerFlowLib/Energy & Power Systems/Hydraulic/Hydraulic Load  fileslct=off  filename=HydraulicLoad.mat  filedir=C:\Users\mwillms4\Dropbox\School\Graduate\Research\PowerFlow Development\PowerFlow Summer 2013\PropertyTables\HydraulicLoad.mat  var_struct=HydraulicLoad  h_load=B_737 - ailerons
  Hydraulic Load2 : PowerFlowLib/Energy & Power Systems/Hydraulic/Hydraulic Load  fileslct=off  filename=HydraulicLoad.mat  filedir=C:\Users\mwillms4\Dropbox\School\Graduate\Research\PowerFlow Development\PowerFlow Summer 2013\PropertyTables\HydraulicLoad.mat  var_struct=HydraulicLoad  h_load=B_737 - elevator
  Hydraulic Load3 : PowerFlowLib/Energy & Power Systems/Hydraulic/Hydraulic Load  fileslct=off  filename=HydraulicLoad.mat  filedir=C:\Users\mwillms4\Dropbox\School\Graduate\Research\PowerFlow Development\PowerFlow Summer 2013\PropertyTables\HydraulicLoad.mat  var_struct=HydraulicLoad  h_load=B_737 - landing_gear
  Hydraulic Load4 : PowerFlowLib/Energy & Power Systems/Hydraulic/Hydraulic Load  fileslct=off  filename=HydraulicLoad.mat  filedir=C:\Users\mwillms4\Dropbox\School\Graduate\Research\PowerFlow Development\PowerFlow Summer 2013\PropertyTables\HydraulicLoad.mat  var_struct=HydraulicLoad  h_load=B_737 - thrust_rev
  Hydraulic Load5 : PowerFlowLib/Energy & Power Systems/Hydraulic/Hydraulic Load  fileslct=off  filename=HydraulicLoad.mat  filedir=C:\Users\mwillms4\Dropbox\School\Graduate\Research\PowerFlow Development\PowerFlow Summer 2013\PropertyTables\HydraulicLoad.mat  var_struct=HydraulicLoad  h_load=B_737 - rudder
  Hydraulic Load6 : PowerFlowLib/Energy & Power Systems/Hydraulic/Hydraulic Load  fileslct=off  filename=HydraulicLoad.mat  filedir=C:\Users\mwillms4\Dropbox\School\Graduate\Research\PowerFlow Development\PowerFlow Summer 2013\PropertyTables\HydraulicLoad.mat  var_struct=HydraulicLoad  h_load=B_737 - ailerons
  Hydraulic Load7 : PowerFlowLib/Energy & Power Systems/Hydraulic/Hydraulic Load  fileslct=off  filename=HydraulicLoad.mat  filedir=C:\Users\mwillms4\Dropbox\School\Graduate\Research\PowerFlow Development\PowerFlow Summer 2013\PropertyTables\HydraulicLoad.mat  var_struct=HydraulicLoad  h_load=B_737 - elevator
  Hydraulic Load8 : PowerFlowLib/Energy & Power Systems/Hydraulic/Hydraulic Load  fileslct=off  filename=HydraulicLoad.mat  filedir=C:\Users\mwillms4\Dropbox\School\Graduate\Research\PowerFlow Development\PowerFlow Summer 2013\PropertyTables\HydraulicLoad.mat  var_struct=HydraulicLoad  h_load=B_737 - landing_gear
  Hydraulic Load9 : PowerFlowLib/Energy & Power Systems/Hydraulic/Hydraulic Load  fileslct=off  filename=HydraulicLoad.mat  filedir=C:\Users\mwillms4\Dropbox\School\Graduate\Research\PowerFlow Development\PowerFlow Summer 2013\PropertyTables\HydraulicLoad.mat  var_struct=HydraulicLoad  h_load=B_737 - thrust_rev
  Memory : Memory
  Mux{,1..3} (4 alike) : Mux  Inputs=5
  Scope{,1..4} (5 alike) : Scope
      Scope2 settings: YMin=-330  YMax=-250  SaveName=ScopeData4
      Scope3 settings: SaveName=ScopeData5
      Scope4 settings: SaveName=ScopeData6
  Sinks : Subsystem
  Terminator : Terminator
  Terminator1 : Terminator
  To Workspace1 : ToWorkspace  VariableName=hydload3  SampleTime=10  SaveFormat=Structure With Time
  To Workspace2 : ToWorkspace  VariableName=hydload4  SampleTime=10  SaveFormat=Structure With Time
  Shaft Torque Eng1 : Outport
  wires:
  Bus Selector15/1 -> [flight_phase]  "<Mssn_phase>"
  Mission/1 -> Bus Selector15/1
  Constant3/1 -> Engine Driven Pump/3  "Pressure_kPa"
  [Eng_Shaft_RPM] -> Engine Driven Pump/2
  Elec/1 -> Bus Selector1/1
  Bus Selector1/1 -> DC Speed Servo/3(Voltage)  "<Voltage>"
  Engine Driven Pump/2 -> Shaft Torque Eng1/1
  Hydraulic Load/1 -> Bus Selector2/1
  Bypass Valve1/1 -> Hydraulic Load3/1, Hydraulic Load4/1, Hydraulic Load2/1, Hydraulic Load1/1, Hydraulic Load/1
  Hydraulic Load1/2 -> Mux1/2
  Hydraulic Load2/2 -> Mux1/3
  Hydraulic Load1/1 -> Bus Selector3/1
  Hydraulic Load2/1 -> Bus Selector4/1
  Bus Selector3/1 -> Mux/2  "<mdot_kgps>"
  Bus Selector2/1 -> Mux/1  "<mdot_kgps>"
  Bus Selector4/1 -> Mux/3  "<mdot_kgps>"
  Mux/1 -> [return_sysB2]
  [flight_phase] -> Hydraulic Load/2, Hydraulic Load1/2, Hydraulic Load3/2, Hydraulic Load4/2, Hydraulic Load2/2
  Hydraulic Load3/1 -> Bus Selector6/1
  Hydraulic Load4/1 -> Bus Selector7/1
  Hydraulic Load4/2 -> Mux1/5
  Hydraulic Load3/2 -> Mux1/4
  Bus Selector6/1 -> Mux/4  "<mdot_kgps>"
  Bus Selector7/1 -> Mux/5  "<mdot_kgps>"
  Hydraulic Load/2 -> Mux1/1
  Mux1/1 -> To Workspace2/1
  Hydraulic Load5/1 -> Bus Selector5/1
  Bypass Valve2/1 -> Hydraulic Load9/1, Hydraulic Load8/1, Hydraulic Load7/1, Hydraulic Load6/1, Hydraulic Load5/1
  Hydraulic Load6/2 -> Mux3/2
  Hydraulic Load7/2 -> Mux3/3
  Hydraulic Load6/1 -> Bus Selector8/1
  Hydraulic Load7/1 -> Bus Selector9/1
  Bus Selector8/1 -> Mux2/2  "<mdot_kgps>"
  Bus Selector5/1 -> Mux2/1  "<mdot_kgps>"
  Bus Selector9/1 -> Mux2/3  "<mdot_kgps>"
  Mux2/1 -> [return_sysA2]
  [flight_phase] -> Hydraulic Load9/2, Hydraulic Load8/2, Hydraulic Load5/2, Hydraulic Load6/2, Hydraulic Load7/2
  Hydraulic Load8/1 -> Bus Selector10/1
  Hydraulic Load9/1 -> Bus Selector11/1
  Hydraulic Load9/2 -> Mux3/5
  Hydraulic Load8/2 -> Mux3/4
  Bus Selector10/1 -> Mux2/4  "<mdot_kgps>"
  Bus Selector11/1 -> Mux2/5  "<mdot_kgps>"
  Hydraulic Load5/2 -> Mux3/1
  Mux3/1 -> To Workspace1/1
  Engine Driven Pump/1 -> Bypass Valve1/1
  Electric Driven Pump/1 -> Bus Selector12/1, Bypass Valve2/1
  [return_sysA2] -> Bypass Valve2/2
  [return_sysB2] -> Bypass Valve1/2
  Constant1/1 -> Electric Driven Pump/3
  Bypass Valve2/2 -> [bypass_elec_pump3]
  [bypass_elec_pump3] -> Bootstrap Reservoir/2(Bypass Return)
  Bootstrap Reservoir/1(Fluid Conditions) -> Scope4/1, Electric Driven Pump/1
  Bus Selector12/1 -> Gain/1, Scope/1  "<pres_kPa>"
  Bus Selector12/2 -> [mdot_out3]  "<mdot_kgps>"
  DC Speed Servo/4(Ploss) -> [Motor_PLoss]
  [Motor_PLoss] -> Sinks/1("Motor PLoss ")
  DC Speed Servo/2(i_load) -> [Hyd_DC_Motor_Load1]
  [Hyd_DC_Motor_Load1] -> Sinks/2(Motor Current Load)
  Bootstrap Reservoir1/1(Fluid Conditions) -> Engine Driven Pump/1, Bus Selector13/1
  Bus Selector13/1 -> Scope1/1, [Hyd_Fluid_High_Pres4]  "<pres_kPa>"
  Bus Selector13/2 -> [mdot_out4]  "<mdot_kgps>"
  [return_sysA2] -> Bootstrap Reservoir/4(Return)
  [return_sysB2] -> Bootstrap Reservoir1/4(Return)
  [mdot_out3] -> Bootstrap Reservoir/3(mdot_out)
  Bypass Valve1/2 -> [bypass_eng_pump4]
  [bypass_eng_pump4] -> Bootstrap Reservoir1/2(Bypass Return)
  [mdot_out4] -> Bootstrap Reservoir1/3(mdot_out)
  [Hyd_Fluid_High_Pres3] -> Bootstrap Reservoir/1(Piston Pressure)
  [Hyd_Fluid_High_Pres4] -> Memory/1
  Constant2/1 -> Bus Creator/1  "Fuel"
  Bus Selector14/1 -> [Eng_Shaft_RPM]  "<Fuel>"
  Bus Creator/1 -> Bus Selector14/1
  DC Speed Servo/3(T_em) -> Terminator1/1
  Sinks/1(Out1) -> Terminator/1
  Electric Driven Pump/2 -> [Electric_Pump_Torque_Load2]
  Constant4/1 -> DC Speed Servo/2(Speed_ref (RPM))
  [Electric_Pump_Torque_Load2] -> DC Speed Servo/1(T_load (Nm)), Scope2/1
  DC Speed Servo/1(w_m) -> Scope3/1, Electric Driven Pump/2, [DC_Motor_RPM2]
  Gain/1 -> [Hyd_Fluid_High_Pres3]
  Memory/1 -> Bootstrap Reservoir1/1(Piston Pressure)

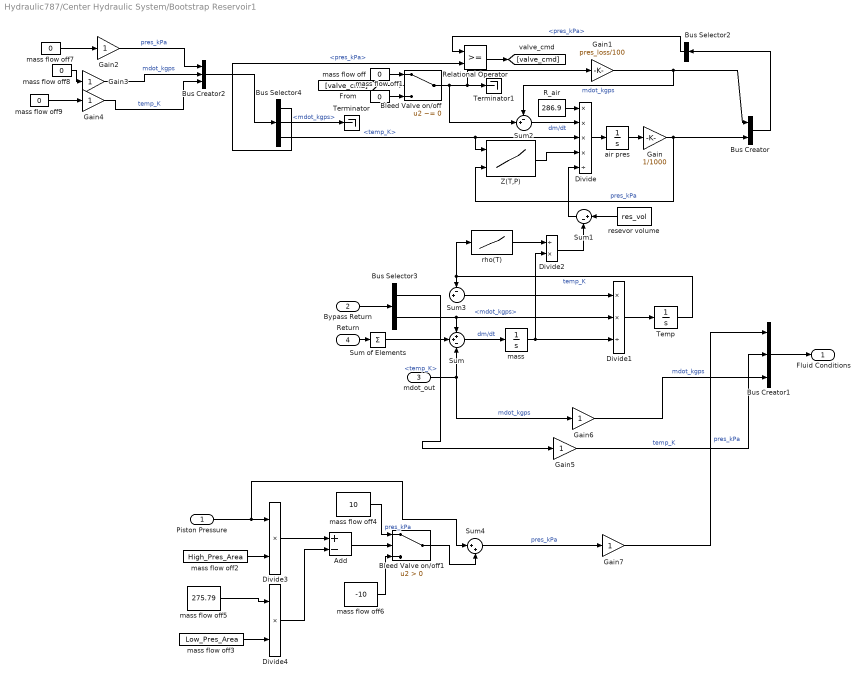
== system Hydraulic787/Center Hydraulic System/Bootstrap Reservoir1 ==
  Piston Pressure : Inport
  Bypass Return : Inport  Port=2
  mdot_out : Inport  Port=3
  Return : Inport  Port=4
  Add : Sum  Inputs=+-
  Bleed Valve on/off : Switch  Criteria=u2 ~= 0  ZeroCross=off
  Bleed Valve on/off1 : Switch  Criteria=u2 > Threshold  ZeroCross=off
  Bus Creator : BusCreator  Inputs=2
  Bus Creator1 : BusCreator  Inputs=3
  Bus Creator2 : BusCreator  Inputs=3
  Bus Selector2 : BusSelector  OutputSignals=pres_kPa
  Bus Selector3 : BusSelector  OutputSignals=temp_K,mdot_kgps
  Bus Selector4 : BusSelector  OutputSignals=pres_kPa,mdot_kgps,temp_K
  Divide : Product  Inputs=****/
  Divide1 : Product  Inputs=**/
  Divide2 : Product  Inputs=/*
  Divide3 : Product  Inputs=**
  Divide4 : Product  Inputs=**
  Gain : Gain  Gain=1/1000
  Gain1 : Gain  Gain=pres_loss/100
  Gain{2..7} (6 alike) : Gain
  R_air : Constant  Value=286.9
  Relational Operator : RelationalOperator  OutDataTypeStr=boolean
  Sum : Sum  Inputs=++-
  Sum of Elements : Sum  Inputs=+
  Sum1 : Sum  Inputs=|+-
  Sum2 : Sum  Inputs=-+|
  Sum3 : Sum  Inputs=-+|
  Sum4 : Sum  Inputs=|++
  Temp : Integrator  InitialCondition=T_init  LimitOutput=on  LowerSaturationLimit=eps
  Terminator : Terminator
  Terminator1 : Terminator
  Z(T,P) : Lookup_n-D  BreakpointsForDimension1=AirProp.T2  BreakpointsForDimension2=AirProp.P2  Table=AirProp.Z  RndMeth=Simplest  InputSameDT=on
  air pres : Integrator  InitialCondition=P_init*1000
  mass : Integrator  InitialCondition=mass_init  LimitOutput=on  LowerSaturationLimit=eps
  mass flow off{,1,7..9} (5 alike) : Constant  Value=0
  mass flow off2 : Constant  Value=High_Pres_Area
  mass flow off3 : Constant  Value=Low_Pres_Area
  mass flow off4 : Constant  Value=10
  mass flow off5 : Constant  Value=275.79
  mass flow off6 : Constant  Value=-10
  resevor volume : Constant  Value=res_vol
  rho(T) : Lookup_n-D  NumberOfTableDimensions=1  BreakpointsForDimension1=HydProp.T  Table=HydProp.rho_T  RndMeth=Simplest  InputSameDT=on
  Fluid Conditions : Outport
  wires:
  Piston Pressure/1 -> Sum4/1, Divide3/1
  mass flow off1/1 -> Bleed Valve on/off/3
  Divide2/1 -> Sum1/2
  rho(T)/1 -> Divide2/1
  Sum of Elements/1 -> Sum/2
  Return/1 -> Sum of Elements/1
  Bus Selector3/1 -> Gain5/1  "<temp_K>"
  Temp/1 -> rho(T)/1, Sum3/1  "temp_K"
  Sum3/1 -> Divide1/1
  Divide1/1 -> Temp/1
  mass/1 -> Divide1/3, Divide2/2
  Bus Creator1/1 -> Fluid Conditions/1
  [valve_cmd] -> Bleed Valve on/off/2
  Relational Operator/1 -> [valve_cmd]
  mass flow off/1 -> Bleed Valve on/off/1
  Bus Selector2/1 -> Relational Operator/1  "<pres_kPa>"
  Bus Selector4/1 -> Relational Operator/2  "<pres_kPa>"
  Bleed Valve on/off/1 -> Terminator1/1, Gain1/1, Sum2/2
  Bus Selector4/2 -> Terminator/1  "<mdot_kgps>"
  Sum2/1 -> Divide/2  "dm/dt"
  Bus Creator/1 -> Bus Selector2/1
  Gain1/1 -> Sum2/1, Bus Creator/1  "mdot_kgps"
  Gain/1 -> Bus Creator/2, Z(T,P)/2  "pres_kPa"
  Sum1/1 -> Divide/5
  resevor volume/1 -> Sum1/1
  air pres/1 -> Gain/1
  Divide/1 -> air pres/1
  Z(T,P)/1 -> Divide/4
  R_air/1 -> Divide/1
  Bus Selector4/3 -> Divide/3, Z(T,P)/1  "<temp_K>"
  Sum/1 -> mass/1  "dm/dt"
  mdot_out/1 -> Gain6/1, Sum/3  "mdot_kgps"
  Bus Selector3/2 -> Sum/1, Divide1/2  "<mdot_kgps>"
  Bypass Return/1 -> Bus Selector3/1
  mass flow off2/1 -> Divide3/2
  mass flow off3/1 -> Divide4/2
  mass flow off5/1 -> Divide4/1
  Divide4/1 -> Add/2
  Divide3/1 -> Add/1
  Add/1 -> Bleed Valve on/off1/2
  mass flow off6/1 -> Bleed Valve on/off1/3
  Bleed Valve on/off1/1 -> Sum4/2
  mass flow off4/1 -> Bleed Valve on/off1/1  "pres_kPa"
  Bus Creator2/1 -> Bus Selector4/1
  mass flow off9/1 -> Gain4/1
  mass flow off8/1 -> Gain3/1
  mass flow off7/1 -> Gain2/1
  Gain2/1 -> Bus Creator2/1  "pres_kPa"
  Gain4/1 -> Bus Creator2/3  "temp_K"
  Gain3/1 -> Bus Creator2/2  "mdot_kgps"
  Gain6/1 -> Bus Creator1/3  "mdot_kgps"
  Gain5/1 -> Bus Creator1/2  "temp_K"
  Sum4/1 -> Gain7/1  "pres_kPa"
  Gain7/1 -> Bus Creator1/1  "pres_kPa"

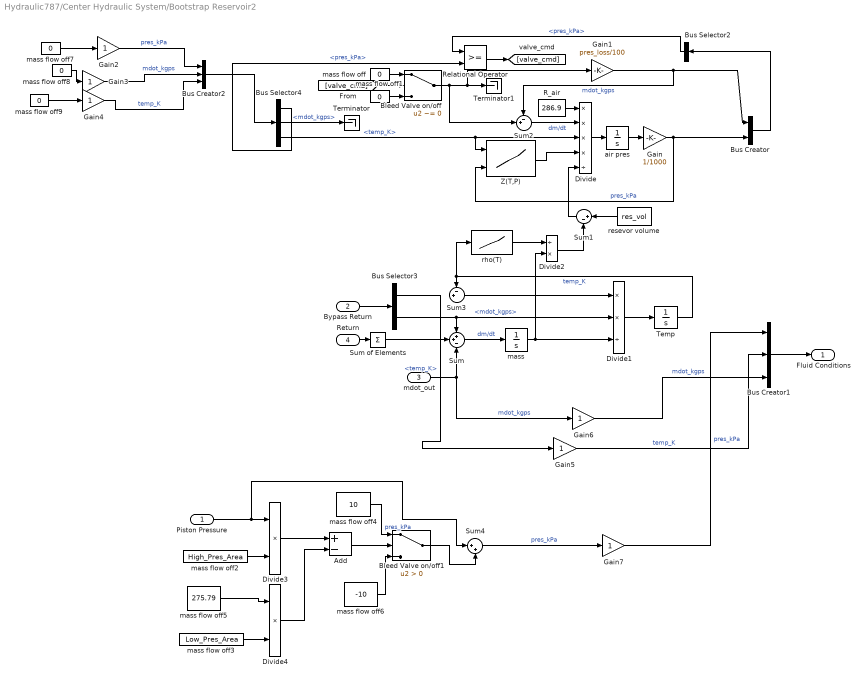
== system Hydraulic787/Center Hydraulic System/Bootstrap Reservoir2 ==
  Piston Pressure : Inport
  Bypass Return : Inport  Port=2
  mdot_out : Inport  Port=3
  Return : Inport  Port=4
  Add : Sum  Inputs=+-
  Bleed Valve on/off : Switch  Criteria=u2 ~= 0  ZeroCross=off
  Bleed Valve on/off1 : Switch  Criteria=u2 > Threshold  ZeroCross=off
  Bus Creator : BusCreator  Inputs=2
  Bus Creator1 : BusCreator  Inputs=3
  Bus Creator2 : BusCreator  Inputs=3
  Bus Selector2 : BusSelector  OutputSignals=pres_kPa
  Bus Selector3 : BusSelector  OutputSignals=temp_K,mdot_kgps
  Bus Selector4 : BusSelector  OutputSignals=pres_kPa,mdot_kgps,temp_K
  Divide : Product  Inputs=****/
  Divide1 : Product  Inputs=**/
  Divide2 : Product  Inputs=/*
  Divide3 : Product  Inputs=**
  Divide4 : Product  Inputs=**
  Gain : Gain  Gain=1/1000
  Gain1 : Gain  Gain=pres_loss/100
  Gain{2..7} (6 alike) : Gain
  R_air : Constant  Value=286.9
  Relational Operator : RelationalOperator  OutDataTypeStr=boolean
  Sum : Sum  Inputs=++-
  Sum of Elements : Sum  Inputs=+
  Sum1 : Sum  Inputs=|+-
  Sum2 : Sum  Inputs=-+|
  Sum3 : Sum  Inputs=-+|
  Sum4 : Sum  Inputs=|++
  Temp : Integrator  InitialCondition=T_init  LimitOutput=on  LowerSaturationLimit=eps
  Terminator : Terminator
  Terminator1 : Terminator
  Z(T,P) : Lookup_n-D  BreakpointsForDimension1=AirProp.T2  BreakpointsForDimension2=AirProp.P2  Table=AirProp.Z  RndMeth=Simplest  InputSameDT=on
  air pres : Integrator  InitialCondition=P_init*1000
  mass : Integrator  InitialCondition=mass_init  LimitOutput=on  LowerSaturationLimit=eps
  mass flow off{,1,7..9} (5 alike) : Constant  Value=0
  mass flow off2 : Constant  Value=High_Pres_Area
  mass flow off3 : Constant  Value=Low_Pres_Area
  mass flow off4 : Constant  Value=10
  mass flow off5 : Constant  Value=275.79
  mass flow off6 : Constant  Value=-10
  resevor volume : Constant  Value=res_vol
  rho(T) : Lookup_n-D  NumberOfTableDimensions=1  BreakpointsForDimension1=HydProp.T  Table=HydProp.rho_T  RndMeth=Simplest  InputSameDT=on
  Fluid Conditions : Outport
  wires:
  Piston Pressure/1 -> Sum4/1, Divide3/1
  mass flow off1/1 -> Bleed Valve on/off/3
  Divide2/1 -> Sum1/2
  rho(T)/1 -> Divide2/1
  Sum of Elements/1 -> Sum/2
  Return/1 -> Sum of Elements/1
  Bus Selector3/1 -> Gain5/1  "<temp_K>"
  Temp/1 -> rho(T)/1, Sum3/1  "temp_K"
  Sum3/1 -> Divide1/1
  Divide1/1 -> Temp/1
  mass/1 -> Divide1/3, Divide2/2
  Bus Creator1/1 -> Fluid Conditions/1
  [valve_cmd] -> Bleed Valve on/off/2
  Relational Operator/1 -> [valve_cmd]
  mass flow off/1 -> Bleed Valve on/off/1
  Bus Selector2/1 -> Relational Operator/1  "<pres_kPa>"
  Bus Selector4/1 -> Relational Operator/2  "<pres_kPa>"
  Bleed Valve on/off/1 -> Terminator1/1, Gain1/1, Sum2/2
  Bus Selector4/2 -> Terminator/1  "<mdot_kgps>"
  Sum2/1 -> Divide/2  "dm/dt"
  Bus Creator/1 -> Bus Selector2/1
  Gain1/1 -> Sum2/1, Bus Creator/1  "mdot_kgps"
  Gain/1 -> Bus Creator/2, Z(T,P)/2  "pres_kPa"
  Sum1/1 -> Divide/5
  resevor volume/1 -> Sum1/1
  air pres/1 -> Gain/1
  Divide/1 -> air pres/1
  Z(T,P)/1 -> Divide/4
  R_air/1 -> Divide/1
  Bus Selector4/3 -> Divide/3, Z(T,P)/1  "<temp_K>"
  Sum/1 -> mass/1  "dm/dt"
  mdot_out/1 -> Gain6/1, Sum/3  "mdot_kgps"
  Bus Selector3/2 -> Sum/1, Divide1/2  "<mdot_kgps>"
  Bypass Return/1 -> Bus Selector3/1
  mass flow off2/1 -> Divide3/2
  mass flow off3/1 -> Divide4/2
  mass flow off5/1 -> Divide4/1
  Divide4/1 -> Add/2
  Divide3/1 -> Add/1
  Add/1 -> Bleed Valve on/off1/2
  mass flow off6/1 -> Bleed Valve on/off1/3
  Bleed Valve on/off1/1 -> Sum4/2
  mass flow off4/1 -> Bleed Valve on/off1/1  "pres_kPa"
  Bus Creator2/1 -> Bus Selector4/1
  mass flow off9/1 -> Gain4/1
  mass flow off8/1 -> Gain3/1
  mass flow off7/1 -> Gain2/1
  Gain2/1 -> Bus Creator2/1  "pres_kPa"
  Gain4/1 -> Bus Creator2/3  "temp_K"
  Gain3/1 -> Bus Creator2/2  "mdot_kgps"
  Gain6/1 -> Bus Creator1/3  "mdot_kgps"
  Gain5/1 -> Bus Creator1/2  "temp_K"
  Sum4/1 -> Gain7/1  "pres_kPa"
  Gain7/1 -> Bus Creator1/1  "pres_kPa"

== system Hydraulic787/Center Hydraulic System/DC Speed Servo ==
  T_load (Nm) : Inport
  Speed_ref (RPM) : Inport  Port=2
  Voltage : Inport  Port=3
  DC Machine : Subsystem
  Fcn : Fcn  Expr=u(1)/(u(2)+0.1)
  Gain2 : Gain  Gain=60/(2*pi)
  Mux : Mux  Inputs=2
  PID Controller : simulink/Continuous/PID Controller  Controller=PID  TimeDomain=Continuous-time  SampleTime=1  IntegratorMethod=Forward Euler  FilterMethod=Forward Euler  Form=Parallel  P=1  I=0.1  D=0  N=100  InitialConditionSource=internal  InitialConditionForIntegrator=0  InitialConditionForFilter=0  ExternalReset=none  LimitOutput=off  UpperSaturationLimit=inf  LowerSaturationLimit=-inf  LinearizeAsGain=on  AntiWindupMode=none  Kb=1  TrackingMode=off  Kt=1  PParamMin=[]  PParamMax=[]  IParamMin=[]  IParamMax=[]  DParamMin=[]  DParamMax=[]  NParamMin=[]  NParamMax=[]  KbParamMin=[]  KbParamMax=[]  KtParamMin=[]  KtParamMax=[]  POutMin=[]  POutMax=[]  IOutMin=[]  IOutMax=[]  DOutMin=[]  DOutMax=[]  NOutMin=[]  NOutMax=[]  KbOutMin=[]  KbOutMax=[]  KtOutMin=[]  KtOutMax=[]  IntegratorOutMin=[]  IntegratorOutMax=[]  FilterOutMin=[]  FilterOutMax=[]  SumOutMin=[]  SumOutMax=[]  SumI1OutMin=[]  SumI1OutMax=[]  SumI2OutMin=[]  SumI2OutMax=[]  SumI3OutMin=[]  SumI3OutMax=[]  SumDOutMin=[]  SumDOutMax=[]  SaturationOutMin=[]  SaturationOutMax=[]  IntegratorContinuousStateAttributes=''  IntegratorStateMustResolveToSignalObject=off  IntegratorRTWStateStorageClass=Auto  FilterContinuousStateAttributes=''  FilterStateMustResolveToSignalObject=off  FilterRTWStateStorageClass=Auto
  Sum : Sum  Inputs=-+|
  Terminator{,1..3} (4 alike) : Terminator
  w_m : Outport
  i_load : Outport  Port=2
  T_em : Outport  Port=3
  Ploss : Outport  Port=4
  wires:
  DC Machine/5(Plosses) -> Ploss/1
  Sum/1 -> PID Controller/1
  Gain2/1 -> Sum/1, w_m/1
  Speed_ref (RPM)/1 -> Sum/2
  T_load (Nm)/1 -> DC Machine/3(Tload)
  DC Machine/6(Te) -> T_em/1
  Mux/1 -> Fcn/1
  DC Machine/3(Pe) -> Mux/1
  Fcn/1 -> i_load/1
  DC Machine/7(Speed) -> Gain2/1
  Voltage/1 -> DC Machine/1(Vf), Mux/2
  PID Controller/1 -> DC Machine/2(Va)
  DC Machine/1(If) -> Terminator/1
  DC Machine/2(Ia) -> Terminator1/1
  DC Machine/4(Pm) -> Terminator2/1
  DC Machine/8(theta) -> Terminator3/1
